simulink model "Problem3"  (R2021a)
settings: Solver=VariableStepAuto  StartTime=0.0  StopTime=10.0  RelTol=1e-3
model workspace (MAT data in the model file):
  K = 0.1584
  k = 0.5792
settings Model: ParameterArgumentNames=K,k  OrderedModelArguments=off  Creator=Nida  LastModifiedBy=Nida

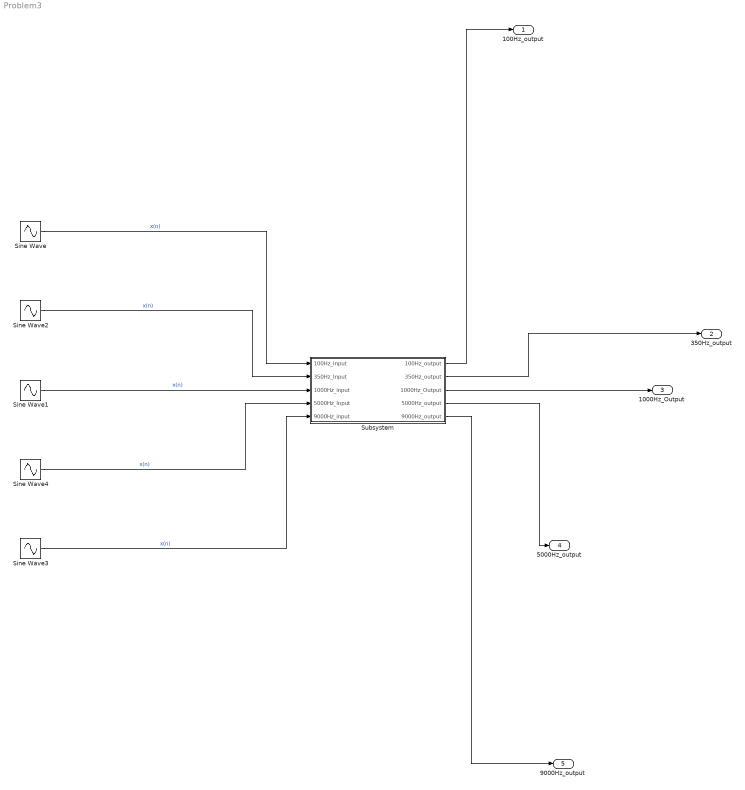
== system Problem3 ==
  Sine Wave{,1..4} (5 alike) : Sin  SampleTime=0
  Subsystem : Subsystem
  100Hz_output : Outport
  350Hz_output : Outport  Port=2
  1000Hz_Output : Outport  Port=3
  5000Hz_output : Outport  Port=4
  9000Hz_output : Outport  Port=5
  wires:
  Sine Wave/1 -> Subsystem/1(100Hz_Input)  "x(n)"
  Sine Wave2/1 -> Subsystem/2(350Hz_Input)  "x(n)"
  Sine Wave1/1 -> Subsystem/3(1000Hz_input)  "x(n)"
  Sine Wave4/1 -> Subsystem/4(5000Hz_Input)  "x(n)"
  Sine Wave3/1 -> Subsystem/5(9000Hz_input)  "x(n)"
  Subsystem/1(100Hz_output) -> 100Hz_output/1
  Subsystem/2(350Hz_output) -> 350Hz_output/1
  Subsystem/3(1000Hz_Output) -> 1000Hz_Output/1
  Subsystem/4(5000Hz_output) -> 5000Hz_output/1
  Subsystem/5(9000Hz_output) -> 9000Hz_output/1

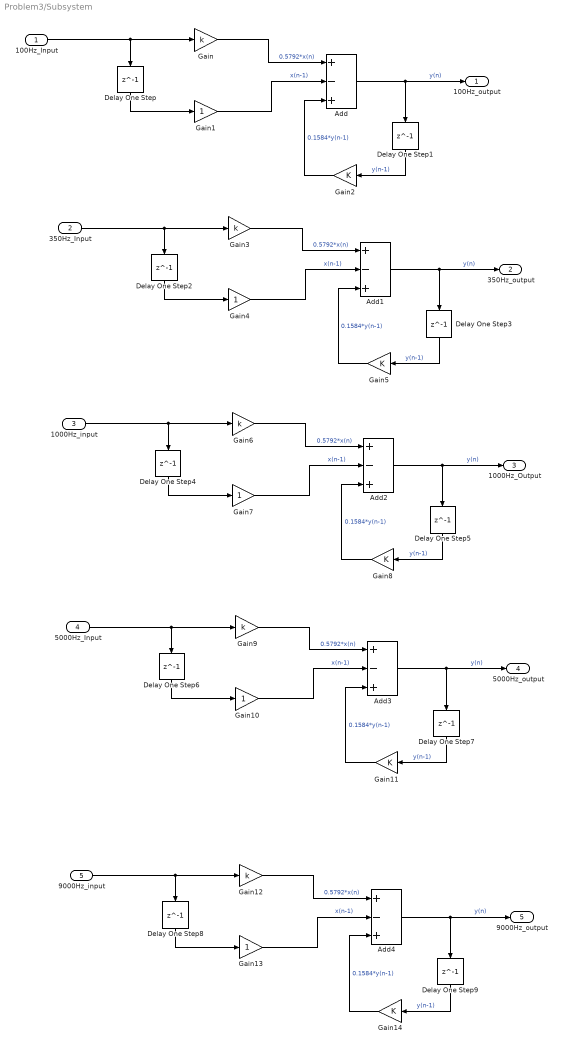
== system Problem3/Subsystem ==
  100Hz_Input : Inport
  350Hz_Input : Inport  Port=2
  1000Hz_input : Inport  Port=3
  5000Hz_Input : Inport  Port=4
  9000Hz_input : Inport  Port=5
  Add{,1..4} (5 alike) : Sum  Inputs=+-+
  Delay One Step{,1..9} (10 alike) : Delay  DelayLength=1
  Gain{,3,6,9,12} (5 alike) : Gain  Gain=k
  Gain{1,4,7,10,13} (5 alike) : Gain
  Gain{2,5,8,11,14} (5 alike) : Gain  Gain=K
  100Hz_output : Outport
  350Hz_output : Outport  Port=2
  1000Hz_Output : Outport  Port=3
  5000Hz_output : Outport  Port=4
  9000Hz_output : Outport  Port=5
  wires:
  9000Hz_input/1 -> Delay One Step8/1, Gain12/1
  Delay One Step6/1 -> Gain10/1
  100Hz_Input/1 -> Delay One Step/1, Gain/1
  Add/1 -> 100Hz_output/1, Delay One Step1/1  "y(n)"
  Delay One Step8/1 -> Gain13/1
  Delay One Step4/1 -> Gain7/1
  Gain10/1 -> Add3/2  "x(n-1)"
  Add3/1 -> 5000Hz_output/1, Delay One Step7/1  "y(n)"
  Add1/1 -> 350Hz_output/1, Delay One Step3/1  "y(n)"
  Gain2/1 -> Add/3  "0.1584*y(n-1)"
  Gain5/1 -> Add1/3  "0.1584*y(n-1)"
  Gain1/1 -> Add/2  "x(n-1)"
  Delay One Step9/1 -> Gain14/1  "y(n-1)"
  350Hz_Input/1 -> Delay One Step2/1, Gain3/1
  Delay One Step2/1 -> Gain4/1
  Gain3/1 -> Add1/1  "0.5792*x(n)"
  Gain11/1 -> Add3/3  "0.1584*y(n-1)"
  Delay One Step3/1 -> Gain5/1  "y(n-1)"
  Gain4/1 -> Add1/2  "x(n-1)"
  Delay One Step1/1 -> Gain2/1  "y(n-1)"
  Gain/1 -> Add/1  "0.5792*x(n)"
  Gain14/1 -> Add4/3  "0.1584*y(n-1)"
  Gain7/1 -> Add2/2  "x(n-1)"
  Delay One Step5/1 -> Gain8/1  "y(n-1)"
  Delay One Step/1 -> Gain1/1
  Delay One Step7/1 -> Gain11/1  "y(n-1)"
  Add2/1 -> 1000Hz_Output/1, Delay One Step5/1  "y(n)"
  1000Hz_input/1 -> Delay One Step4/1, Gain6/1
  Gain9/1 -> Add3/1  "0.5792*x(n)"
  5000Hz_Input/1 -> Delay One Step6/1, Gain9/1
  Gain6/1 -> Add2/1  "0.5792*x(n)"
  Gain8/1 -> Add2/3  "0.1584*y(n-1)"
  Add4/1 -> 9000Hz_output/1, Delay One Step9/1  "y(n)"
  Gain12/1 -> Add4/1  "0.5792*x(n)"
  Gain13/1 -> Add4/2  "x(n-1)"
